simulink model "ex7"  (R2018b)
settings: Solver=VariableStepAuto  StartTime=0.0  StopTime=10.0  RelTol=1e-3
libraries: fuzblock x1
settings Model: Creator=Fraxinus  LastModifiedBy=Fraxinus

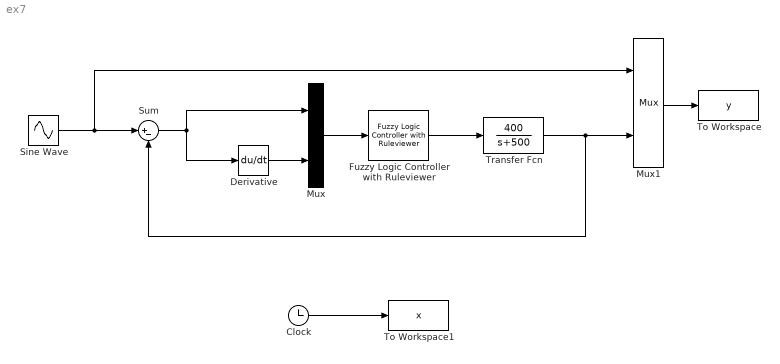
== system ex7 ==
  Clock : Clock
  Derivative : Derivative
  Fuzzy Logic Controller with Ruleviewer : fuzblock/Fuzzy Logic  Controller  with Ruleviewer  fismatrix=myFLC  Ts=2
  Mux : Mux  Inputs=2
  Mux1 : Mux  Inputs=2
  Sine Wave : Sin  Amplitude=0.5  Frequency=10  SampleTime=0
  Sum : Sum  Inputs=|+-
  To Workspace : ToWorkspace  VariableName=y  SaveFormat=Timeseries  SampleTime=-1
  To Workspace1 : ToWorkspace  VariableName=x  SaveFormat=Timeseries  SampleTime=-1
  Transfer Fcn : TransferFcn  Numerator=[400]  Denominator=[1 500]
  wires:
  Mux/1 -> Fuzzy Logic Controller with Ruleviewer/1
  Derivative/1 -> Mux/2
  Fuzzy Logic Controller with Ruleviewer/1 -> Transfer Fcn/1
  Sine Wave/1 -> Mux1/1, Sum/1
  Mux1/1 -> To Workspace/1
  Transfer Fcn/1 -> Sum/2, Mux1/2
  Sum/1 -> Derivative/1, Mux/1
  Clock/1 -> To Workspace1/1
